simulink model "Robot_KinematicsSim_2019b1"  (R2020b)
settings: Solver=VariableStepAuto  StartTime=0.0  StopTime=1000  RelTol=1e-3  EnableMultiTasking=on
model workspace (MAT data in the model file):
  Ts = 0.01
  Xmax = 500
  Ymax = 500
values from neighbouring files (symbols this model uses):
  animation_update_interval = C*h_fixed    [setup.m]
  enable_CG_trace = 1    [setup.m]
  enable_rearAxle_trace = 0    [setup.m]
  plotAxisLimitMode = 0    [setup.m]
  plotAxisLimits = plotAxisLimits    [graphical_development.m]    (also in setup.m = [-3 5 -3 6]*3)
  save_anim_frames = 0    [setup.m]
  vehicle_length = 5    [setup.m]
  vehicle_width = 2    [setup.m]
undefined symbols (not defined in the file or in its folder): datetime, DiscIntNeverNeededParam
libraries: arduinolib x21, simulink x4, pid_lib x2
(part 2 of 2)

== matlab function Robot_KinematicsSim_2019b1/Vehicle Simulation Subsystem /MATLAB Function ==
  data: pwm input; pwm1 input; y output; direction input; direction1 input; y1 output
function [y,y1] = fcn(pwm, pwm1, direction,direction1)
    if(direction == 1 && direction1 == 0)
       y= pwm;
       y1= pwm1;
    elseif(direction == 0 && direction1 == 0) 
        y=-pwm;
        y1= pwm1;
        
    else
        y=pwm;
        y1= -pwm1;
    end
        
        
    end

== matlab function Robot_KinematicsSim_2019b1/Vehicle Simulation Subsystem /Vechicle's Path /MATLAB Function  ==
  data: theta input; x_prime output; Vr input; Vl input; y_prime output
function [x_prime,y_prime] = VehiclesPath(theta, Vr, Vl)

Vavg = (Vr+Vl)/2;
x_prime = Vavg*sind(theta);
y_prime = Vavg*cosd(theta);

== matlab function Robot_KinematicsSim_2019b1/Vehicle Simulation Subsystem2/Vechicle's Path /MATLAB Function  ==
  data: theta input; x_prime output; Vr input; Vl input; y_prime output
function [x_prime,y_prime] = VehiclesPath(theta, Vr, Vl)

Vavg = (Vr+Vl)/2;
x_prime = Vavg*sind(theta);
y_prime = Vavg*cosd(theta);

== matlab function Robot_KinematicsSim_2019b1/MATLAB Function ==
  data: lat1 input; a output; lon1 input; lat2 input; lon2 input; c output; n input; s output; ss input


function [a,c,s]=haversine(lat1,lon1,lat2,lon2,n,ss)
% HAVERSINE_FORMULA.AWK - converted from AWK

s=0;
coder.extrinsic('writematrix');
coder.extrinsic('readmatrix');
coder.extrinsic('disp');
%data=[0 0;lat1 lon1;lat2 lon2];
    %filename = 'C:\Users\Omen\Desktop\a.xlsx';
    
    %writematrix(data,filename);
    T = readmatrix('C:\Users\Omen\Desktop\route.xlsx');
    
    sz=0;
    sz=size(T,1);
    y=0;
    y1=0;
    y2=0;
    y3=0;
    y4=0;
  
 if(n<(sz-1))
     n=double(n)+1; 
 end
 
    
    y=T((n+2),1);
    y1=T((n+1),1);
    y2=T((n+2),2);
    y3=T((n+1),2);
    dlat = radians(y-y1);
    dlon = radians(y2-y3);
    lat1 = radians(y1);
    lat2 = radians(y);
    
    a=0;
    a=T((n+1),3);
    
     a1 = (sin(dlat./2)).^2 + cos(lat1) .* cos(lat2) .* (sin(dlon./2)).^2;
    c = 2 .* asin(sqrt(a1)).*6372.8;
    s=ss+c;   
   
    


 
 
end
function rad = radians(degree) 
% degrees to radians
        rad = degree .* pi / 180;
end

== stateflow chart Robot_KinematicsSim_2019b1/CruiseControlAndAutomaticBraking1 ==
  note: Requirements -
      |
      | § The robot should run as fast as it can. (Cruise Mode)
      | § So it should be programmed so that If it sees other robots
      | that are moving, it should slow down to its pace but still keep moving. (Follow Leader)
      | § If it sees other robots that are stationary, it should come to
      | a stop and wait for them to get out of its way. (Brake)
  state CruiseMode
    en,du:
    RWCommand = 10;
    LWCommand = 10;
  state FollowLeader
    state Start
    state DistanceDecreasing
      state Strat2
      state GradualDecrease
        state SlowFall
          en,du:
          RWCommand = ...
          RWCommandUD+...
          0.05*(IRData-IRDataUD);
          LWCommand = ...
          RWCommandUD+...
          0.05*(IRData-IRDataUD);
        state Decelerate
          en, du:
          RWCommand = ...
          RWCommandUD-...
          slope*Ts;
          LWCommand = ...
          LWCommandUD-...
          slope*Ts;
        (default) -> SlowFall
        SlowFall -> Decelerate : after(1,sec)
      state SharpDecrease
        en,du:
        RWCommand = ...
        RWCommandUD-slope*Ts;
        LWCommand = ...
        LWCommandUD-slope*Ts;
      (default) -> Strat2
      Strat2 -> (junction 133)
      (junction 133) -> GradualDecrease [order 2] : [IRData - IRDataUD>-DisTh]
      (junction 133) -> SharpDecrease [order 1] : [IRData - IRDataUD<-DisTh]
    state DistanceConstant
      en,du:
      RWCommand = RWCommandUD;
      LWCommand = LWCommandUD;
    state DistanceIncreasing
      state Start3
      state GradualIncrease
        state SlowRise
          en,du:
          RWCommand = ...
          RWCommandUD+...
          0.05*(IRData-IRDataUD);
          LWCommand = ...
          RWCommandUD+...
          0.05*(IRData-IRDataUD);
        state Accelerate
          en, du:
          RWCommand = ...
          RWCommandUD+...
          slope*Ts;
          LWCommand = ...
          LWCommandUD+...
          slope*Ts;
        (default) -> SlowRise
        SlowRise -> Accelerate : after(1,sec)
      state SharpIncrease
        en,du:
        RWCommand = ...
        RWCommandUD+slope*Ts;
        LWCommand = ...
        LWCommandUD+slope*Ts;
      (default) -> Start3
      Start3 -> (junction 145)
      (junction 145) -> GradualIncrease [order 2] : [IRData - IRDataUD>-DisTh]
      (junction 145) -> SharpIncrease [order 1] : [IRData - IRDataUD>DisTh]
    (default) -> Start
    Start -> (junction 120)
    (junction 120) -> DistanceIncreasing [order 2] : [IRData-IRDataUD> IRTh]
    (junction 120) -> DistanceDecreasing [order 1] : [IRData - IRDataUD <-IRTh]
    (junction 120) -> DistanceConstant [order 3] : [abs(IRData-IRDataUD) <IRTh]
    DistanceDecreasing -> DistanceConstant [order 1] : [abs(IRData-IRDataUD) <IRTh]
    DistanceIncreasing -> DistanceConstant [order 2] : [abs(IRData-IRDataUD) <IRTh]
    DistanceConstant -> DistanceDecreasing [order 1] : [IRData-IRDataUD <-IRTh]
    DistanceConstant -> DistanceIncreasing [order 2] : [IRData-IRDataUD >IRTh]
    DistanceDecreasing -> DistanceIncreasing [order 2] : [IRData-IRDataUD > IRTh]
    DistanceIncreasing -> DistanceDecreasing [order 1] : [IRData-IRDataUD < -IRTh]
  state Brake
    en,du:
    RWCommand = 0	;
    LWCommand = 0;
  (default) -> CruiseMode
  FollowLeader -> CruiseMode [order 1] : [IRData > 50]
  CruiseMode -> FollowLeader : [IRData < 50]
  Brake -> FollowLeader : [IRData >= 20 ]
  FollowLeader -> Brake [order 2] : [IRData < 20]
  data: IRData input; RWCommand output double [0..]; LWCommand output double; IRDataUD input; RWCommandUD input; LWCommandUD input; DisTh input; IRTh input; slope constant double =3.5; Ts constant double =0.01

== matlab function Robot_KinematicsSim_2019b1/Path Navigation1/LW Encoder ticks counter ==
  data: encoder_ticks input; y output; count input; reset input
function y = fcn(encoder_ticks,count,reset)
    
    if (reset==1)
        count=0;
    end
    if (encoder_ticks==1)
        count=count+1;
    end
y = count;

== matlab function Robot_KinematicsSim_2019b1/Path Navigation1/RW Encoder ticks counter ==
  data: encoder_ticks input; y output; count input; reset input
function y = fcn(encoder_ticks,count,reset)
    
    if (reset==1)
        count=0;
    end
    if (encoder_ticks==1)
        count=count+1;
    end
y = count;

== matlab function Robot_KinematicsSim_2019b1/Path Navigation1/Speed Control Logic ==
  settings: updateMethod=DISCRETE
  data: LeftEnc input; LeftMtr output; RightEnc input; RightMtr output; out1 output; out2 output; out3 output; out4 output; PIDVal input; TicksLine input; TicksTurn input; res output; res2 input; res1 output
function [LeftMtr,RightMtr,out1,out2,out3,out4,res,res1] = controlSpeed(LeftEnc,RightEnc,PIDVal,TicksLine,TicksTurn,res2)
%#codegen
persistent RobotMotion %Variable to keep track of robot state (i.e move straight or take turn)

if isempty(RobotMotion)
    RobotMotion=1; %Initializing variable to the first robot state 1 (i.e first straight motion).Odd values for straight motion and even values for turn
end

res=0;
out1=0;
out2=0;
out3=0;
out4=0;
res1=res2;
switch RobotMotion
    case {1} %Checking if the robot state is to take turn
        
        %Check if the encoder count is less than required ticks for turn. Since a delay of 1 sample time is required to 
        %reset the encoder value (due to Unit Delay block in the model), the encoder count value exceeds the required 
        %ticks for straight line for one sample time after the robot state changes for taking turn
        
        if(abs(RightEnc)<abs(TicksTurn) && abs(LeftEnc)<abs(TicksTurn))
            LeftMtr=10;
            
            %Same speed is applied to both motors to take turn since the motors are connected in 
            %opposite direction to the robot platform
            RightMtr=10;
            if (TicksTurn>0)
                out1=1;
                out2=0;
                out3=0;
                out4=1;
            else
                out1=0;
                out2=1;
                out3=1;
                out4=0;
            end
            
         %   Reset=0;
        else
            LeftMtr=0;
            RightMtr=0;
            RobotMotion=RobotMotion+1; %Changing the robot state to move straight
            
            res=1; %Making the Reset signal to encoder high to reset the encoder
        end
        
    case {2} %Checking if the robot state is to move straight
        
        %Check if the encoder count is less than required ticks for straight line 
        if(abs(LeftEnc)<=TicksLine && abs(RightEnc)<=TicksLine) 
            
            LeftMtr=10; 
            RightMtr=10;
            out1=1;
            out2=0;
            out3=1;
            out4=0;
            
        else %Encoder count has exceeded the required ticks for straight line
            
            LeftMtr=0; 
            RightMtr=0;
            RobotMotion=RobotMotion+1; %Changing the robot state to take turn
            res=1; %Making the Reset signal to encoder high to reset the encoder
        end    
        
    otherwise %Robot state is at a value greater than 8 (i.e it has completed tracing the square path)
        
        res1=res2+1;
        LeftMtr=0;
        RightMtr=0;
        RobotMotion=1;
        res=1;
        
end
end

== matlab function Robot_KinematicsSim_2019b1/Vehicle Simulation Subsystem 1/MATLAB Function To enable reversing the Left Motors  ==
  data: pwm input; LWCommand output; direction input
function LWCommand = fcn(pwm, direction)
    if(direction == 1)
       LWCommand= pwm;
    else 
        LWCommand=-pwm;
        
    end

== matlab function Robot_KinematicsSim_2019b1/Vehicle Simulation Subsystem 1/Vechicle's Path /MATLAB Function  ==
  data: theta input; x_prime output; Vr input; Vl input; y_prime output
function [x_prime,y_prime] = VehiclesPath(theta, Vr, Vl)

Vavg = (Vr+Vl)/2;
x_prime = -Vavg*sind(theta);
y_prime = Vavg*cosd(theta);
